simulink model "test_sch"  (R2018a)
settings: Solver=VariableStepAuto  StartTime=0.0  StopTime=20  RelTol=1e-3
values from neighbouring files (symbols this model uses):
  A1 = 1    [Uklad_Wersja_Laczna.m]    (also in Uklad_wersja_Liniowa.m; Uklad_wersja_Nieliniowa.m; test.m)
  A2 = 1    [Uklad_Wersja_Laczna.m]    (also in Uklad_wersja_Liniowa.m; Uklad_wersja_Nieliniowa.m; test.m)
  Aw1 = 0.1*A1    (= 0.1)    [Uklad_Wersja_Laczna.m]    (also in Uklad_wersja_Liniowa.m; Uklad_wersja_Nieliniowa.m; test.m)
  Aw2 = 0.2*A2    (= 0.2)    [Uklad_Wersja_Laczna.m]    (also in Uklad_wersja_Liniowa.m; Uklad_wersja_Nieliniowa.m; test.m)
  dfew1 = 0.1*fwe_max    [Uklad_Wersja_Laczna.m]    (also in Uklad_wersja_Liniowa.m = 0; Uklad_wersja_Nieliniowa.m = 1; test.m = 1)
  fwe1 = f(i)    [Uklad_Wersja_Laczna.m]    (also in Uklad_wersja_Liniowa.m = 1; Uklad_wersja_Nieliniowa.m = 1; test.m = 0)
  g = 10    [Uklad_Wersja_Laczna.m]    (also in Uklad_wersja_Liniowa.m = 9.81; Uklad_wersja_Nieliniowa.m = 9.81; test.m = 9.81)
  h10 = 1    [Uklad_Wersja_Laczna.m]    (also in Uklad_wersja_Liniowa.m = 3; Uklad_wersja_Nieliniowa.m = 5.09683995923; test.m = 0.6)
  h20 = 1    [Uklad_Wersja_Laczna.m]    (also in Uklad_wersja_Liniowa.m = 2; Uklad_wersja_Nieliniowa.m = 1.27420998981; test.m = 2)
  steptime_1 = 3    [Uklad_Wersja_Laczna.m]    (also in Uklad_wersja_Liniowa.m = 0; Uklad_wersja_Nieliniowa.m; test.m)
settings Model: Creator=johnb  LastModifiedBy=johnb

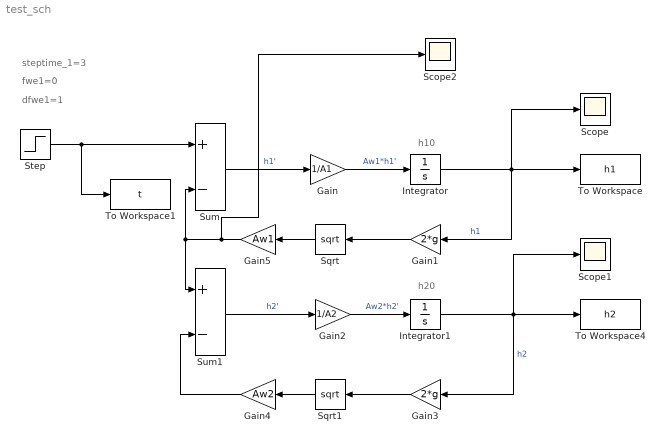
== system test_sch ==
  note: dfwe1=1
  note: fwe1=0
  note: steptime_1=3
  note: h20
  note: h10
  Gain : Gain  Gain=1/A1
  Gain1 : Gain  Gain=2*g
  Gain2 : Gain  Gain=1/A2
  Gain3 : Gain  Gain=2*g
  Gain4 : Gain  Gain=Aw2
  Gain5 : Gain  Gain=Aw1
  Integrator : Integrator  InitialCondition=h10
  Integrator1 : Integrator  InitialCondition=h20
  Scope : Scope
  Scope1 : Scope
  Scope2 : Scope
  Sqrt : Sqrt  SaturateOnIntegerOverflow=on
  Sqrt1 : Sqrt  SaturateOnIntegerOverflow=on
  Step : Step  Time=steptime_1  Before=fwe1  After=dfew1+fwe1  SampleTime=0
  Sum : Sum  Inputs=+-
  Sum1 : Sum  Inputs=+-
  To Workspace : ToWorkspace  VariableName=h1  SampleTime=-1
  To Workspace1 : ToWorkspace  VariableName=t  SaveFormat=Timeseries  SampleTime=-1
  To Workspace4 : ToWorkspace  VariableName=h2  SampleTime=-1
  wires:
  Step/1 -> To Workspace1/1, Sum/1
  Gain/1 -> Integrator/1  "Aw1*h1'"
  Sum/1 -> Gain/1  "h1'"
  Integrator/1 -> Gain1/1, To Workspace/1, Scope/1  "h1"
  Gain1/1 -> Sqrt/1
  Sqrt/1 -> Gain5/1
  Gain3/1 -> Sqrt1/1
  Integrator1/1 -> Gain3/1, Scope1/1, To Workspace4/1  "h2"
  Gain2/1 -> Integrator1/1  "Aw2*h2'"
  Sum1/1 -> Gain2/1  "h2'"
  Sqrt1/1 -> Gain4/1
  Gain5/1 -> Scope2/1, Sum1/1, Sum/2
  Gain4/1 -> Sum1/2
